simulink model "seMM1QueuingSys"  (R2024a)
settings: Solver=VariableStepAuto  StartTime=0.0  StopTime=100  RelTol=1e-3  EnableMultiTasking=on
undefined symbols (not defined in the file): m, n
libraries: simulink x2
settings Model: Creator=The MathWorks, Inc.  LastModifiedBy=kaspe
settings SolverCC: AlgebraicLoopSolver=TrustRegion
settings DataIOCC: LimitDataPoints=on  SaveFormat=Array  ReturnWorkspaceOutputs=off
settings OptimizationCC: LifeSpan=inf
settings DebuggingCC: UnconnectedInputMsg=warning  UnconnectedOutputMsg=warning  UnconnectedLineMsg=warning  AllowSymbolicDim=off  SFUnexpectedBacktrackingDiag=warning  SFNoUnconditionalDefaultTransitionDiag=warning  SFExecutionAtInitializationDiag=none  ArithmeticOperatorsInVariantConditions=warning
settings ModelReferenceCC: EnableRefExpFcnMdlSchedulingChecks=on  PropagateSignalLabelsOutOfModel=off
settings SFSimCC: SimUseLocalCustomCode=off  CustomCodeUndefinedFunction=UseInterfaceOnly
settings RTWCC: RTWUseLocalCustomCode=off  GPUComputeCapability=3.5  DLArmComputeVersion=19.05
settings CodeAppCC: StateflowObjectComments=on
settings GRTTargetCC: TargetLangStandard=C89/C90 (ANSI)
settings ConfigComp: CovMetricSettings=dw  CovSaveCumulativeToWorkspaceVar=on  CovSaveSingleToWorkspaceVar=on  CovExternalEMLEnable=off  CovSFcnEnable=off

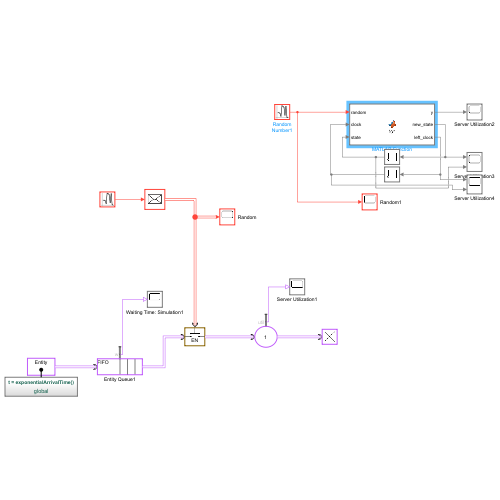
[thumbnail: Simulink's stored preview of the top-level diagram]
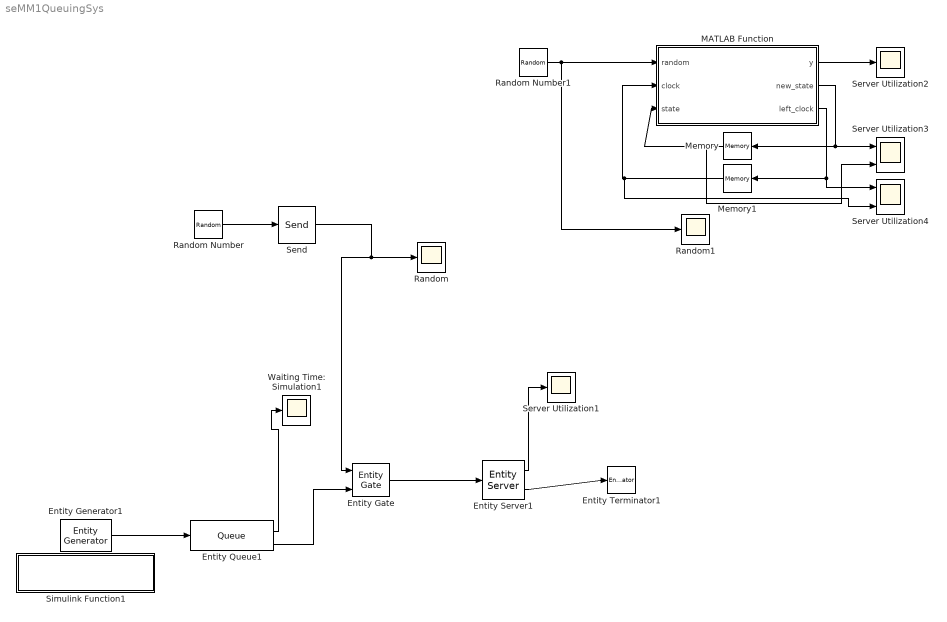
== system seMM1QueuingSys ==
  Entity Gate : EntityGate  InputPortMessageModes=m,m  OutputPortMessageModes=m
  Entity Generator1 : EntityGenerator  OutputPortMessageModes=m  TimeSource=MATLAB action  IntergenerationTimeAction=dt = exponentialArrivalTime();  EntityType=Structured  EntityTypeName=Entity
  Entity Queue1 : Queue  InputPortMessageModes=m  OutputPortMessageModes=n,m  Capacity=Inf  AverageWait=on
      settings: OutputPortMap=o2,o5
  Entity Server1 : EntityServer  InputPortMessageModes=m  OutputPortMessageModes=n,m  Capacity=1  ServiceTimeSource=MATLAB action  ServiceTimeAction=|  Utilization=on
      | % Exponential service time with rate 1
      | mean = 1;
      | dt   = -mean * log(1 - rand());
      settings: OutputPortMap=o5,o9
  Entity Terminator1 : EntityTerminator  InputPortMessageModes=m
  MATLAB Function : MATLAB Function  TreatAsAtomicUnit=on
  Memory : Memory
  Memory1 : Memory
  Random : Scope
  Random Number : RandomNumber  Variance=0.125  Seed=10  SampleTime=10
  Random Number1 : RandomNumber  Variance=0.125  Seed=11  SampleTime=10
  Random1 : Scope
  Send : Send  OutputPortMessageModes=m
  Server Utilization1 : Scope
  Server Utilization2 : Scope
  Server Utilization3 : Scope  NumInputPorts=2
  Server Utilization4 : Scope  NumInputPorts=2
  Simulink Function1 : Subsystem  TreatAsAtomicUnit=on
  Waiting Time: Simulation1 : Scope
  wires:
  Entity Generator1/1 -> Entity Queue1/1
  Entity Queue1/1 -> Waiting Time: Simulation1/1
  Entity Gate/1 -> Entity Server1/1
  Random Number/1 -> Send/1
  Send/1 -> Entity Gate/1, Random/1
  Entity Server1/1 -> Server Utilization1/1
  Entity Server1/2 -> Entity Terminator1/1
  Entity Queue1/2 -> Entity Gate/2
  Random Number1/1 -> Random1/1, MATLAB Function/1(random)
  MATLAB Function/1(y) -> Server Utilization2/1
  MATLAB Function/2(new_state) -> Server Utilization3/1, Memory/1
  Memory/1 -> Server Utilization3/2, MATLAB Function/3(state)
  MATLAB Function/3(left_clock) -> Server Utilization4/1, Memory1/1
  Memory1/1 -> Server Utilization4/2, MATLAB Function/2(clock)

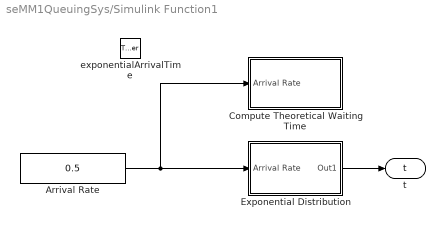
== system seMM1QueuingSys/Simulink Function1 ==
  exponentialArrivalTime : TriggerPort  TriggerType=function-call  IsSimulinkFunction=on  FunctionName=exponentialArrivalTime  VariantControl=Variant
  Arrival Rate : Constant  Value=0.5  SampleTime=-1
  Compute Theoretical Waiting Time : Subsystem
  Exponential Distribution : Subsystem
  t : ArgOut  DisableCoverage=on  ArgumentName=t
  wires:
  Arrival Rate/1 -> Compute Theoretical Waiting Time/1(Arrival Rate), Exponential Distribution/1(Arrival Rate)
  Exponential Distribution/1(Out1) -> t/1

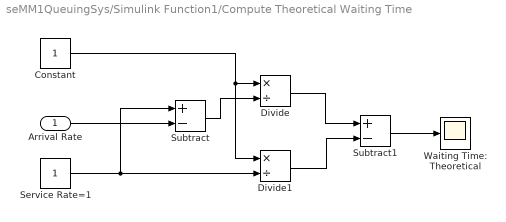
== system seMM1QueuingSys/Simulink Function1/Compute Theoretical Waiting Time ==
  Arrival Rate : Inport
  Constant : Constant
  Divide : Product  Inputs=*/
  Divide1 : Product  Inputs=*/
  Service Rate=1 : Constant
  Subtract : Sum  Inputs=+-
  Subtract1 : Sum  Inputs=+-
  Waiting Time: Theoretical : Scope
  wires:
  Arrival Rate/1 -> Subtract/2
  Subtract1/1 -> Waiting Time: Theoretical/1
  Divide1/1 -> Subtract1/2
  Divide/1 -> Subtract1/1
  Subtract/1 -> Divide/2
  Constant/1 -> Divide1/1, Divide/1
  Service Rate=1/1 -> Subtract/1, Divide1/2

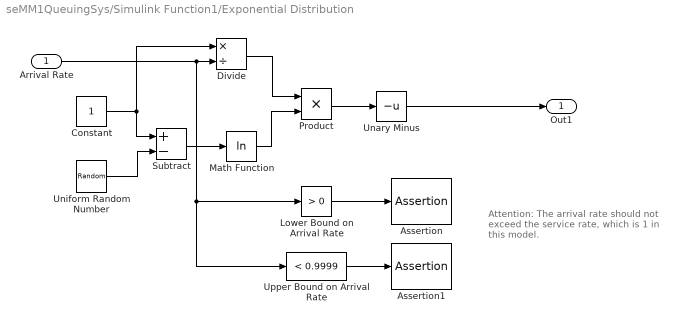
== system seMM1QueuingSys/Simulink Function1/Exponential Distribution ==
  note: Attention: The arrival rate
      | should not exceed the service
      | rate, which is 1 in this model.
  Arrival Rate : Inport
  Assertion : Assertion
  Assertion1 : Assertion
  Constant : Constant
  Divide : Product  Inputs=*/
  Lower Bound on Arrival Rate : simulink/Logic and Bit Operations/Compare To Constant  relop=>  const=0  OutDataTypeStr=uint8  ZeroCross=off
  Math Function : Math  Operator=log  SignedPower=on
  Product : Product  RndMeth=Zero
  Subtract : Sum  Inputs=+-
  Unary Minus : UnaryMinus
  Uniform Random Number : UniformRandomNumber  Minimum=0  Seed=12345
  "Upper Bound on Arrival Rate " : simulink/Logic and Bit Operations/Compare To Constant  relop=<  const=0.9999  OutDataTypeStr=uint8  ZeroCross=off
  Out1 : Outport
  wires:
  Arrival Rate/1 -> Divide/2, Lower Bound on Arrival Rate/1, "Upper Bound on Arrival Rate "/1
  Unary Minus/1 -> Out1/1
  Product/1 -> Unary Minus/1
  Math Function/1 -> Product/2
  Divide/1 -> Product/1
  Constant/1 -> Divide/1, Subtract/1
  Uniform Random Number/1 -> Subtract/2
  Lower Bound on Arrival Rate/1 -> Assertion/1
  "Upper Bound on Arrival Rate "/1 -> Assertion1/1
  Subtract/1 -> Math Function/1

== matlab function seMM1QueuingSys/MATLAB Function ==
  data: random input; y output; clock input; state input; new_state output; left_clock output
function [y, new_state, left_clock] = fcn(random, clock, state)

    if random < 0 && state == 0
        new_state = 1;
        left_clock = randi([1, 5]);
        %left_clock = 5;
        y = -1;
    elseif state == 1 
        if clock == 0
            y = 1;
            new_state = 0;
            left_clock = 0;
        else
            left_clock = clock - 1;
            new_state = state;
            y = -1;
        end
    else
        y = 1;
        new_state = 0;
        left_clock = 0;
    end  
end
